simulink model "singularity_in_continuous"  (R2015a)
settings: Solver=ode45  StartTime=0.0  StopTime=10.0  RelTol=1e-3
libraries: simulink x4
settings Model: Creator=shafiul  LastModifiedBy=shafiul

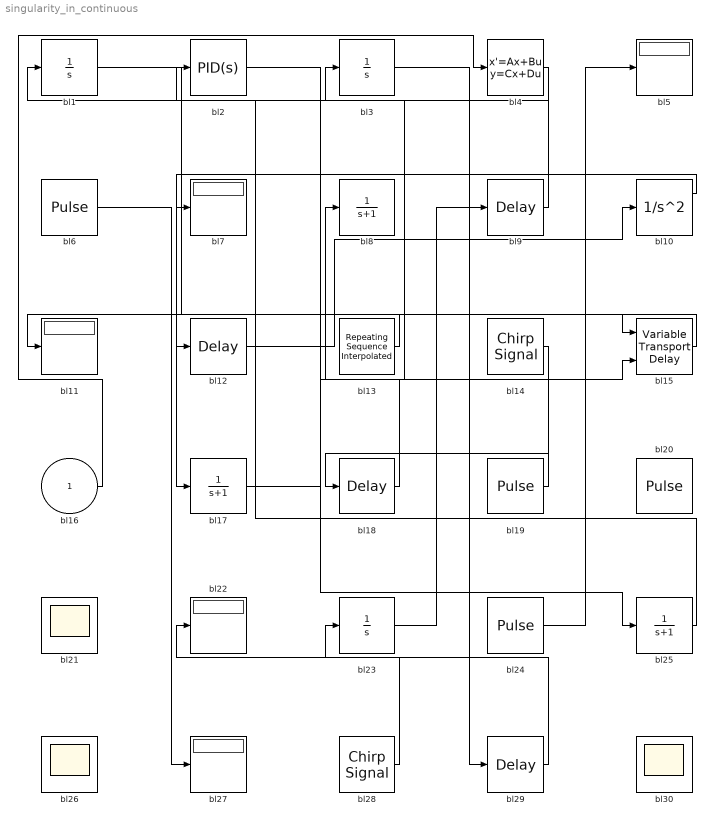
== system singularity_in_continuous ==
  bl16 : Inport
  bl1 : Integrator  LimitOutput=on  UpperSaturationLimit=1  LowerSaturationLimit=0
  bl10 : SecondOrderIntegrator
  bl{5,7,11,22,27} (5 alike) : Display
  bl12 : TransportDelay  InitialOutput=1
  bl13 : simulink/Sources/Repeating Sequence Interpolated  OutValues=[3 1 4 2 1].'  TimeValues=[0 0.1 0.5 0.6 1].'  LookUpMeth=Interpolation-Use End Values  tsamp=0.01  OutMin=[]  OutMax=[]  OutDataTypeStr=double  OutputDataTypeScalingMode=double  OutDataType=fixdt(0,8)  OutScaling=2^-10
  bl14 : simulink/Sources/Chirp Signal  f1=0.1  T=100  f2=1
  bl15 : VariableTransportDelay  VariableDelayType=Variable transport delay  MaximumDelay=10  InitialOutput=3
  bl17 : TransferFcn  Denominator=[1 1]
  bl18 : TransportDelay  InitialOutput=3
  bl{6,19..20,24} (4 alike) : DiscretePulseGenerator  PulseType=Time based  Period=10  PulseWidth=5
  bl2 : simulink/Continuous/PID Controller  Controller=PID  TimeDomain=Continuous-time  SampleTime=-1  IntegratorMethod=Forward Euler  FilterMethod=Forward Euler  Form=Parallel  UseFilter=on  ControllerParametersSource=internal  P=1  I=1  D=0  N=100  InitialConditionSource=internal  InitialConditionForIntegrator=0  InitialConditionForFilter=0  ExternalReset=none  LimitOutput=off  UpperSaturationLimit=inf  LowerSaturationLimit=-inf  LinearizeAsGain=on  AntiWindupMode=none  Kb=1  TrackingMode=off  Kt=1  PParamMin=[]  PParamMax=[]  IParamMin=[]  IParamMax=[]  DParamMin=[]  DParamMax=[]  NParamMin=[]  NParamMax=[]  KbParamMin=[]  KbParamMax=[]  KtParamMin=[]  KtParamMax=[]  POutMin=[]  POutMax=[]  IOutMin=[]  IOutMax=[]  DOutMin=[]  DOutMax=[]  NOutMin=[]  NOutMax=[]  KbOutMin=[]  KbOutMax=[]  KtOutMin=[]  KtOutMax=[]  IntegratorOutMin=[]  IntegratorOutMax=[]  FilterOutMin=[]  FilterOutMax=[]  SumOutMin=[]  SumOutMax=[]  SumI1OutMin=[]  SumI1OutMax=[]  SumI2OutMin=[]  SumI2OutMax=[]  SumI3OutMin=[]  SumI3OutMax=[]  SumDOutMin=[]  SumDOutMax=[]  SaturationOutMin=[]  SaturationOutMax=[]  IntegratorContinuousStateAttributes=''  IntegratorStateMustResolveToSignalObject=off  IntegratorRTWStateStorageClass=Auto  FilterContinuousStateAttributes=''  FilterStateMustResolveToSignalObject=off  FilterRTWStateStorageClass=Auto  DifferentiatorICPrevScaledInput=0  DifferentiatorOutMin=[]  DifferentiatorOutMax=[]
  bl21 : Scope
      settings: Floating=on
  bl23 : Integrator  LimitOutput=on  UpperSaturationLimit=1  LowerSaturationLimit=0
  bl25 : TransferFcn  Denominator=[1 1]
  bl26 : Scope
      settings: Floating=on
  bl28 : simulink/Sources/Chirp Signal  f1=0.1  T=100  f2=1
  bl29 : TransportDelay  InitialOutput=2
  bl3 : Integrator  LimitOutput=on  UpperSaturationLimit=1  LowerSaturationLimit=0
  bl30 : Scope
      settings: Floating=on
  bl4 : StateSpace  X0=0
  bl8 : TransferFcn  Denominator=[1 1]
  bl9 : TransportDelay  InitialOutput=3
  wires:
  bl18/1 -> bl8/1
  bl23/1 -> bl9/1
  bl13/1 -> bl11/1
  bl29/1 -> bl22/1
  bl24/1 -> bl5/1
  bl28/1 -> bl23/1
  bl9/1 -> bl1/1
  bl4/1 -> bl17/1
  bl16/1 -> bl4/1
  bl14/1 -> bl18/1
  bl1/1 -> bl15/1
  bl12/1 -> bl10/1
  bl19/1 -> bl3/1
  bl6/1 -> bl27/1
  bl2/1 -> bl25/1
  bl3/1 -> bl29/1
  bl15/1 -> bl12/1
  bl17/1 -> bl15/2
  bl25/1 -> bl2/1
  bl10/1 -> bl7/1
